simulink model "chap10_2sim"  (Simulink 8.1)
settings: Solver=ode45  StartTime=0  StopTime=10  FixedStep=0.0001  RelTol=1e-5
settings Model: Creator=hp  LastModifiedBy=liujk  ExtModeTrigMode=oneshot  ExtModeArmWhenConnect=off
settings DataIOCC: LimitDataPoints=off  SignalLoggingName=sigsOut
settings OptimizationCC: BooleanDataType=off  InitFltsAndDblsToZero=on
settings DebuggingCC: SaveWithParameterizedLinksMsg=none  SignalResolutionControl=TryResolveAllWithWarning  SolverPrmCheckMsg=none  MultiTaskDSMMsg=warning  MultiTaskCondExecSysMsg=none  FcnCallInpInsideContextMsg=EnableAllAsWarning  StrictBusMsg=None
settings HardwareCC: TargetUnknown=on
settings RTWCC: IncludeERTFirstTime=on
settings GRTTargetCC: TargetFcnLib=ansi_tfl_tmw.mat

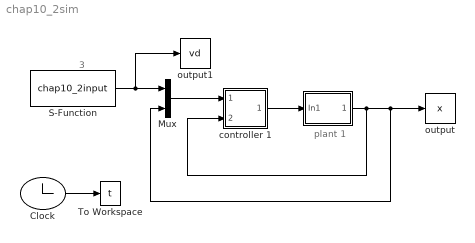
== system chap10_2sim ==
  note: 3
  note: plant 1
  " " : Subsystem
  Clock : Clock
      settings: Decimation=5
  Mux : Mux  Inputs=2
  S-Function : S-Function  FunctionName=chap10_2input  EnableBusSupport=off
  To Workspace : ToWorkspace  VariableName=t  SampleTime=-1
  controller 1 : Subsystem
  output : ToWorkspace  VariableName=x  SampleTime=-1
  output1 : ToWorkspace  VariableName=vd  SampleTime=-1
  wires:
  Clock/1 -> To Workspace/1
  S-Function/1 -> output1/1, Mux/1
  Mux/1 -> controller 1/1(In1)
  " "/1(Out1) -> output/1, Mux/2, controller 1/2(In2)
  controller 1/1(Out2) -> " "/1(In1)

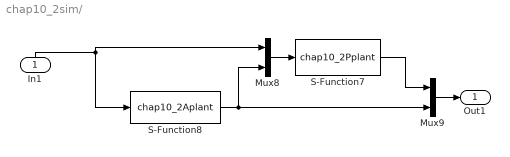
== system chap10_2sim/  ==
  In1 : Inport
  Mux8 : Mux  Inputs=2
  Mux9 : Mux  Inputs=2
  S-Function7 : S-Function  FunctionName=chap10_2Pplant  EnableBusSupport=off
  S-Function8 : S-Function  FunctionName=chap10_2Aplant  EnableBusSupport=off
  Out1 : Outport
  wires:
  S-Function7/1 -> Mux9/1
  S-Function8/1 -> Mux9/2, Mux8/2
  Mux8/1 -> S-Function7/1
  In1/1 -> S-Function8/1, Mux8/1
  Mux9/1 -> Out1/1

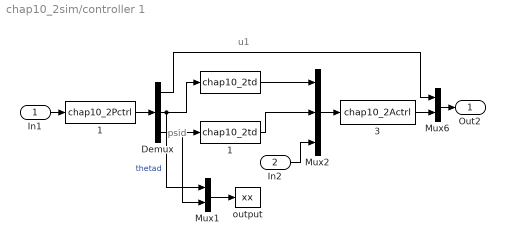
== system chap10_2sim/controller 1 ==
  note: u1
  note: psid
  In1 : Inport
  In2 : Inport  Port=2
  "  " : S-Function  FunctionName=chap10_2td  EnableBusSupport=off
  "    3" : S-Function  FunctionName=chap10_2Actrl  EnableBusSupport=off
  "   1" : S-Function  FunctionName=chap10_2Pctrl  EnableBusSupport=off
  "  1" : S-Function  FunctionName=chap10_2td  EnableBusSupport=off
  Demux : Demux  Outputs=3
  Mux1 : Mux  Inputs=2
  Mux2 : Mux  Inputs=3
  Mux6 : Mux  Inputs=2
  output : ToWorkspace  VariableName=xx  SampleTime=-1
  Out2 : Outport
  wires:
  "   1"/1 -> Demux/1
  Demux/1 -> Mux6/1
  Demux/2 -> "  "/1, Mux1/1  "thetad"
  Demux/3 -> Mux1/2, "  1"/1
  Mux2/1 -> "    3"/1
  In1/1 -> "   1"/1
  "    3"/1 -> Mux6/2
  Mux6/1 -> Out2/1
  In2/1 -> Mux2/3
  "  "/1 -> Mux2/1
  "  1"/1 -> Mux2/2
  Mux1/1 -> output/1
